simulink model "OpAmpFeedback"  (R2021b)
settings: Solver=VariableStepAuto  StartTime=0.0  StopTime=inf  MaxStep=1e-4  RelTol=1e-3
libraries: fl_lib x11, nesl_utility x5, ee_lib x2
settings Model: PacingRate=0.010000  Creator=Work  LastModifiedBy=Work

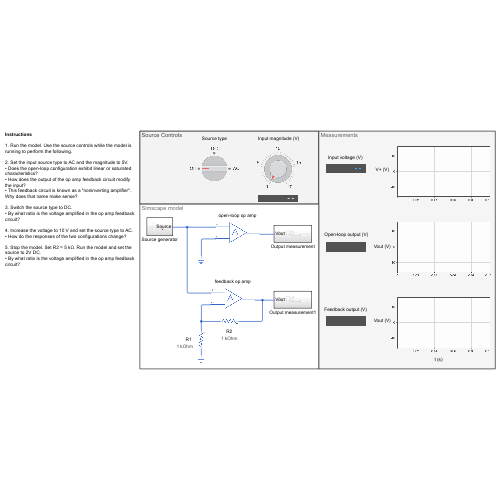
[thumbnail: Simulink's stored preview of the top-level diagram]
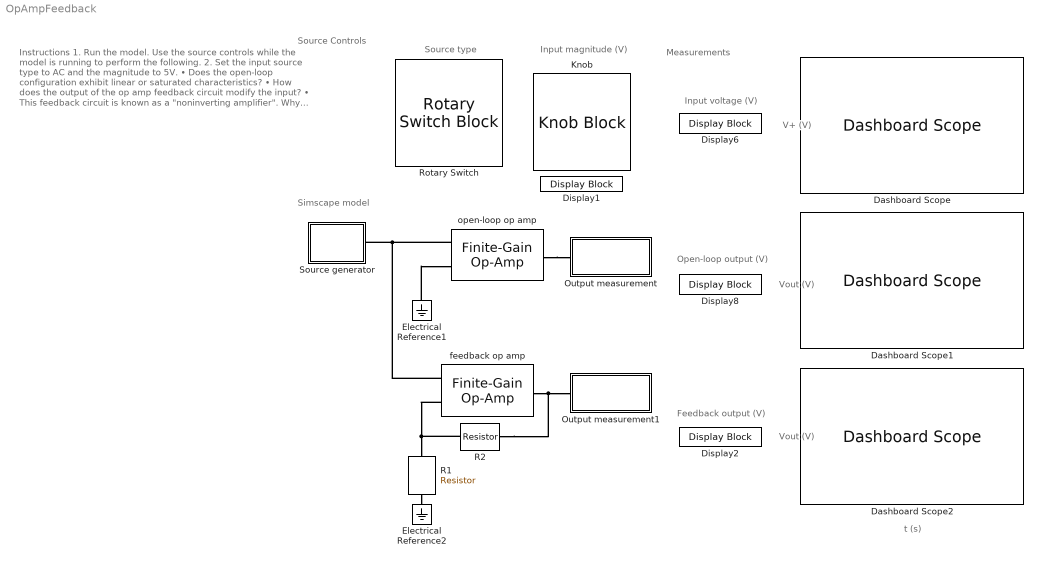
== system OpAmpFeedback ==
  note: V+ (V)
  note: Input magnitude (V)
  note: Source type
  note: Instructions
      |
      | 1. Run the model. Use the source controls while the model is running to perform the following.
      |
      | 2. Set the input source type to AC and the magnitude to 5V.
      | • Does the open-loop configuration exhibit linear or saturated characteristics?
      | • How does the output of the op amp feedback circuit modify the input?
      | • This feedback circuit is known as a "noninverting amplifier". Why does that name make sense?
      |
      | 3. Switch the source type to DC.
      | • By what ratio is the voltage amplified in the op amp feedback circuit?
      |
      | 4. Increase the voltage to 10 V and set the source type to AC.
      | • How do the responses of the two configurations change?
      |
      | 5. Stop the model. Set R2 = 5 k Ω . Run the model and set the source to 2V DC.
      | • By what ratio is the voltage amplified in the op amp feedback circuit?
  note: Source Controls
  note: Measurements
  note: Simscape model
  note: Input voltage (V)
  note: Open-loop output (V)
  note: Feedback output (V)
  note: t (s)
  note: Vout (V)
  note: Vout (V)
  Dashboard Scope : DashboardScope  TimeSpan=0.10000000000000001  Ymin=-16  Ymax=16  ScaleAtStop=off  UpdateMode=Scroll
  Dashboard Scope1 : DashboardScope  TimeSpan=0.10000000000000001  Ymin=-16  Ymax=16  ScaleAtStop=off  UpdateMode=Scroll
  Dashboard Scope2 : DashboardScope  TimeSpan=0.10000000000000001  Ymin=-16  Ymax=16  ScaleAtStop=off  UpdateMode=Scroll
  Display{1..2,6,8} (4 alike) : DisplayBlock  LabelPosition=Hide  Format=Custom  Alignment=Right  Transparency=1  FormatString=%0.4f
  Electrical Reference1 : fl_lib/Electrical/Electrical Elements/Electrical Reference
  Electrical Reference2 : fl_lib/Electrical/Electrical Elements/Electrical Reference
  Knob : KnobBlock  LabelPosition=Hide  ScaleMax=20  TickInterval=5
  Output measurement : Subsystem
  Output measurement1 : Subsystem
  R1 : fl_lib/Electrical/Electrical Elements/Resistor  R=1 kOhm  i_specify=off  i_priority=None  i=0 A  i_nominal_specify=off  i_nominal_unit=A  i_nominal_value=1  v_specify=off  v_priority=None  v=0 V  v_nominal_specify=off  v_nominal_unit=V  v_nominal_value=1
      settings: AttributesFormatString=%<R> %<R_unit>
  R2 : fl_lib/Electrical/Electrical Elements/Resistor  R=1 kOhm  i_specify=off  i_priority=None  i=0 A  i_nominal_specify=off  i_nominal_unit=A  i_nominal_value=1  v_specify=off  v_priority=None  v=0 V  v_nominal_specify=off  v_nominal_unit=V  v_nominal_value=1
      settings: AttributesFormatString=%<R> %<R_unit>
  Rotary Switch : RotarySwitchBlock  LabelPosition=Hide
      settings: Values={{'Off', 'DC', 'AC'}, [0 1 2]}
  Source generator : Subsystem
  feedback op amp : ee_lib/Integrated Circuits/Finite-Gain Op-Amp  A=1e5  Rin=1e6 Ohm  Rout=100 Ohm  Vmin=-15 V  Vmax=15 V  noise_mode=0  v_noise=30e-9 V/Hz^(1/2)  noise_prm=1  i_noise=0.5e-12 A/Hz^(1/2)  ip_noise=0.5e-12 A/Hz^(1/2)  in_noise=0.5e-12 A/Hz^(1/2)  sample_time=1e-3 s  repeatability=1  auto_seed_v=3499211588  auto_seed_ip=3890346746  auto_seed_in=545404223  user_seed_v=0  user_seed_ip=0  user_seed_in=0
      settings: SourceProductBaseCode=PS  InternalSimscapePortConfiguration="{\"Bottom\":[],\"Left\":[{\"id\":\"p\",\"label\":\"+\",\"type\":\"foundation.electrical.electrical\"},{\"id\":\"n\",\"label\":\"-\",\"type\":\"foundation.electrical.electrical\"}],\"Right\":[{\"id\":\"out\",\"label\":\"\",\"type\":\"foundation.electrical.electrical\"}],\"Top\":[]}"
  open-loop op amp : ee_lib/Integrated Circuits/Finite-Gain Op-Amp  A=2e3  Rin=1e6 Ohm  Rout=100 Ohm  Vmin=-15 V  Vmax=15 V  noise_mode=0  v_noise=30e-9 V/Hz^(1/2)  noise_prm=1  i_noise=0.5e-12 A/Hz^(1/2)  ip_noise=0.5e-12 A/Hz^(1/2)  in_noise=0.5e-12 A/Hz^(1/2)  sample_time=1e-3 s  repeatability=1  auto_seed_v=1041471841  auto_seed_ip=230873357  auto_seed_in=1897181789  user_seed_v=0  user_seed_ip=0  user_seed_in=0
      settings: SourceProductBaseCode=PS  InternalSimscapePortConfiguration="{\"Bottom\":[],\"Left\":[{\"id\":\"p\",\"label\":\"+\",\"type\":\"foundation.electrical.electrical\"},{\"id\":\"n\",\"label\":\"-\",\"type\":\"foundation.electrical.electrical\"}],\"Right\":[{\"id\":\"out\",\"label\":\"\",\"type\":\"foundation.electrical.electrical\"}],\"Top\":[]}"
  connections:
  Electrical Reference1/LConn1 -- open-loop op amp/LConn2
  open-loop op amp/LConn1 -- feedback op amp/LConn1 -- Source generator/RConn1
  open-loop op amp/RConn1 -- Output measurement/LConn1
  R1/RConn1 -- Electrical Reference2/LConn1
  feedback op amp/RConn1 -- R2/LConn1 -- Output measurement1/LConn1
  R2/RConn1 -- feedback op amp/LConn2 -- R1/LConn1

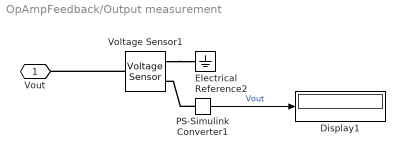
== system OpAmpFeedback/Output measurement ==
  Display1 : Display
  Electrical Reference2 : fl_lib/Electrical/Electrical Elements/Electrical Reference
  PS-Simulink Converter1 : nesl_utility/PS-Simulink Converter  PhysicalDomain=network_engine_domain  SubClassName=ps_output  LeftPortType=input  RightPortType=output  PseudoPeriodic=off  Frequencies=[]  Unit=inherit  AffineConversion=off
      settings: SourceProductBaseCode=PW,SS
  Voltage Sensor1 : fl_lib/Electrical/Electrical Sensors/Voltage Sensor
  Vout : PMIOPort  Side=Left
  wires:
  PS-Simulink Converter1/1 -> Display1/1  "Vout"
  connections:
  Voltage Sensor1/LConn1 -- Vout/RConn1
  Voltage Sensor1/RConn2 -- Electrical Reference2/LConn1
  PS-Simulink Converter1/LConn1 -- Voltage Sensor1/RConn1

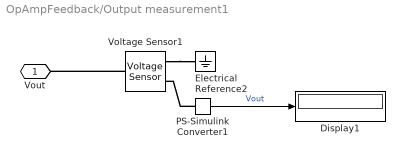
== system OpAmpFeedback/Output measurement1 ==
  Display1 : Display
  Electrical Reference2 : fl_lib/Electrical/Electrical Elements/Electrical Reference
  PS-Simulink Converter1 : nesl_utility/PS-Simulink Converter  PhysicalDomain=network_engine_domain  SubClassName=ps_output  LeftPortType=input  RightPortType=output  PseudoPeriodic=off  Frequencies=[]  Unit=inherit  AffineConversion=off
      settings: SourceProductBaseCode=PW,SS
  Voltage Sensor1 : fl_lib/Electrical/Electrical Sensors/Voltage Sensor
  Vout : PMIOPort  Side=Left
  wires:
  PS-Simulink Converter1/1 -> Display1/1  "Vout"
  connections:
  Voltage Sensor1/LConn1 -- Vout/RConn1
  Voltage Sensor1/RConn2 -- Electrical Reference2/LConn1
  PS-Simulink Converter1/LConn1 -- Voltage Sensor1/RConn1

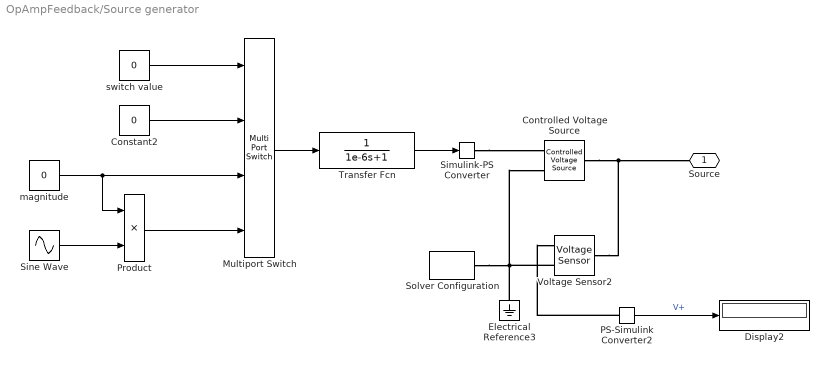
== system OpAmpFeedback/Source generator ==
  Constant2 : Constant  Value=0
  Controlled Voltage Source : fl_lib/Electrical/Electrical Sources/Controlled Voltage Source
  Display2 : Display
  Electrical Reference3 : fl_lib/Electrical/Electrical Elements/Electrical Reference
  Multiport Switch : MultiPortSwitch  DataPortOrder=Zero-based contiguous  zeroidx=on
  PS-Simulink Converter2 : nesl_utility/PS-Simulink Converter  PhysicalDomain=network_engine_domain  SubClassName=ps_output  LeftPortType=input  RightPortType=output  PseudoPeriodic=off  Frequencies=[]  Unit=inherit  AffineConversion=off
      settings: SourceProductBaseCode=PW,SS
  Product : Product
  Simulink-PS Converter : nesl_utility/Simulink-PS Converter  PhysicalDomain=network_engine_domain  SubClassName=ps_input  LeftPortType=input  RightPortType=output  PseudoPeriodic=off  Frequencies=[]  NoiseDistribution=none  NoiseParameters=[]  Unit=1  AffineConversion=off  FilteringAndDerivatives=provide  SimscapeFilterOrder=1  InputFilterTimeConstant=0.001  UdotUserProvided=0
      settings: SourceProductBaseCode=PW,SS
  Sine Wave : Sin  Frequency=2*pi*60  SampleTime=0
  Solver Configuration : nesl_utility/Solver Configuration  PhysicalDomain=network_engine_domain  SubClassName=solver  LeftPortType=input  RightPortType=generic  Tones=[]  Harmonics=[]  SimulateNoise=off  Profile=off  UseLocalSampling=off  EnableSwitchedLinearOptims=on  FrequencyDomain=off  UseCCode=off  RelTol=0.001  AbsTol=1e-06  MinStep=1e-09  ToWorkspace=off  RevertToSquareIcSolve=off  NumHomotopyIterations=100  PhasorMode=off  PhasorModeNumHarmonics=1  DoDC=off  ResidualTolerance=1e-09  UseLocalSolver=off  LocalSolverChoice=NE_BACKWARD_EULER_ADVANCER  LocalSolverSampleTime=0.001  DoFixedCost=off  MaxNonlinIter=3  MaxModeIter=2  ComputeImpulses=off  ImpulseIterations=2  LinearAlgebra=auto  EquationFormulation=NE_TIME_EF  DelaysMemoryBudget=1024  AutomaticFiltering=on  FilteringTimeConstant=0.001  PartitionStorageMethod=AS_NEEDED  PartitionMemoryBudget=1024  PartitionMethod=ROBUST
      settings: SourceProductBaseCode=PW,SS
  Transfer Fcn : TransferFcn  Denominator=[1e-6 1]
  Voltage Sensor2 : fl_lib/Electrical/Electrical Sensors/Voltage Sensor
  magnitude : Constant  Value=0
  switch value : Constant  Value=0
  Source : PMIOPort  Side=Right
  wires:
  PS-Simulink Converter2/1 -> Display2/1  "V+"
  Sine Wave/1 -> Product/2
  magnitude/1 -> Multiport Switch/3, Product/1
  Product/1 -> Multiport Switch/4
  Multiport Switch/1 -> Transfer Fcn/1
  switch value/1 -> Multiport Switch/1
  Constant2/1 -> Multiport Switch/2
  Transfer Fcn/1 -> Simulink-PS Converter/1
  connections:
  Electrical Reference3/LConn1 -- Solver Configuration/RConn1 -- Controlled Voltage Source/RConn2 -- Voltage Sensor2/RConn2
  Controlled Voltage Source/LConn1 -- Voltage Sensor2/LConn1 -- Source/RConn1
  PS-Simulink Converter2/LConn1 -- Voltage Sensor2/RConn1
  Simulink-PS Converter/RConn1 -- Controlled Voltage Source/RConn1
